simulink model "sl_ploop_test"  (R2022a)
settings: Solver=ode15s  StartTime=0.0  StopTime=1  RelTol=1e-3  EnableMultiTasking=on
PreLoadFcn:
  | G = 107.815;
InitFcn:
  | G = 107.815;
libraries: roblocks x1, robotcorelib x1
Description:
  | Test harness for position control loop with
  | trapezoidal trajectory.
  | 
  | Robotics, Vision and Control - 3rd Edition; Section 9.1.7
settings Model: Creator=pic  LastModifiedBy=rpill
settings SolverCC: AlgebraicLoopSolver=TrustRegion  MaxZcPerStep=1
settings DataIOCC: SaveFormat=Array  SignalLoggingSaveFormat=ModelDataLogs  TimeSaveName=t  OutputSaveName=y  OutputOption=SpecifiedOutputTimes  OutputTimes=[0:0.001:1]'
settings OptimizationCC: ExpressionDepthLimit=2147483647  LifeSpan=inf
settings DebuggingCC: UnderspecifiedInitializationDetection=Classic  MergeDetectMultiDrivingBlocksExec=none  SolverPrmCheckMsg=warning  UnconnectedInputMsg=warning  UnconnectedOutputMsg=warning  UnconnectedLineMsg=warning  AllowSymbolicDim=off  StateNameClashWarn=warning  SFUnexpectedBacktrackingDiag=warning  SFNoUnconditionalDefaultTransitionDiag=warning  SFExecutionAtInitializationDiag=none  SFMachineParentedDataDiag=warning  ArithmeticOperatorsInVariantConditions=warning
settings HardwareCC: ProdBitPerPointer=32  ProdBitPerSizeT=32  ProdBitPerPtrDiffT=32  ProdLargestAtomicFloat=None  ProdIntDivRoundTo=Undefined  ProdEndianess=Unspecified  ProdWordSize=32  ProdHWDeviceType=32-bit Generic
settings ModelReferenceCC: PropagateSignalLabelsOutOfModel=off
settings SFSimCC: SimUseLocalCustomCode=off  CustomCodeUndefinedFunction=UseInterfaceOnly
settings RTWCC: RTWUseLocalCustomCode=off
settings CodeAppCC: StateflowObjectComments=on
settings GRTTargetCC: TargetLangStandard=C89/C90 (ANSI)  CombineOutputUpdateFcns=off  GRTInterface=on
settings ConfigComp: CovMetricSettings=dw  CovSaveCumulativeToWorkspaceVar=on  CovSaveSingleToWorkspaceVar=on  CovExternalEMLEnable=off  CovSFcnEnable=off

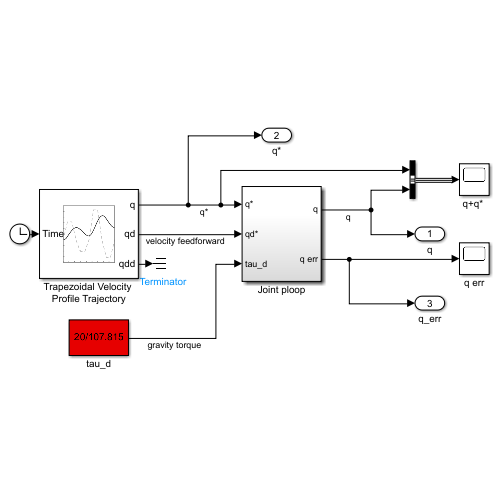
[thumbnail: Simulink's stored preview of the top-level diagram]
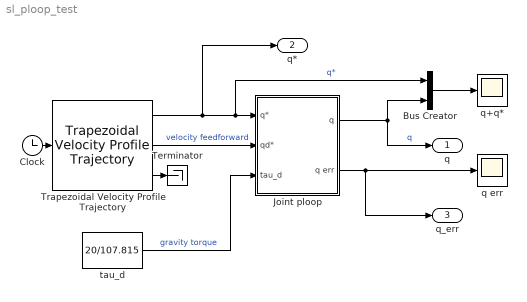
== system sl_ploop_test ==
  Bus Creator : BusCreator  Inputs=2
  Clock : Clock
  Joint ploop : Subsystem
  Terminator : Terminator
  Trapezoidal Velocity Profile Trajectory : robotcorelib/Trapezoidal Velocity Profile Trajectory  WaypointSource=Internal  Waypoints=[0 1]  NumParams=1  Parameter1=End Time  Parameter2=End Time  ParameterSource=Internal  PeakVelocity=[ 2; 2 ]  Acceleration=[ 1; 2 ]  EndTime=[1]  AccelTime=[ 1; 2 ]  SimulateUsing=Interpreted execution
      settings: SourceProductBaseCode=RO,NV,RR,UV
  q err : Scope
  "q+q* " : Scope
  tau_d : Constant  Value=20/107.815
  q : Outport  VectorParamsAs1DForOutWhenUnconnected=off
  q* : Outport  Port=2  VectorParamsAs1DForOutWhenUnconnected=off
  q_err : Outport  Port=3  VectorParamsAs1DForOutWhenUnconnected=off
  wires:
  Joint ploop/1(q) -> Bus Creator/2, q/1  "q"
  Joint ploop/2(q err) -> q_err/1, q err/1
  Trapezoidal Velocity Profile Trajectory/1 -> q*/1, Bus Creator/1, Joint ploop/1(q*)  "q*"
  tau_d/1 -> Joint ploop/3(tau_d)  "gravity torque"
  Trapezoidal Velocity Profile Trajectory/3 -> Terminator/1
  Trapezoidal Velocity Profile Trajectory/2 -> Joint ploop/2(qd*)  "velocity feedforward"
  Bus Creator/1 -> "q+q* "/1
  Clock/1 -> Trapezoidal Velocity Profile Trajectory/1

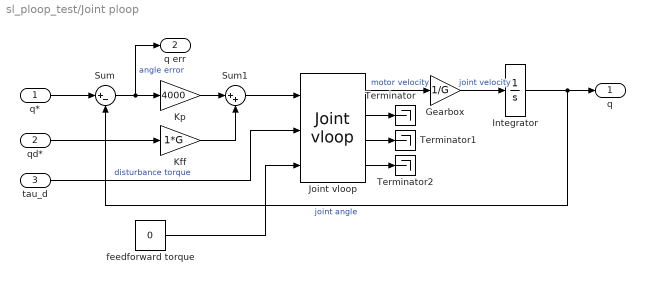
== system sl_ploop_test/Joint ploop ==
  q* : Inport
  qd* : Inport  Port=2
  tau_d : Inport  Port=3
  Gearbox : Gain  Gain=1/G
  Integrator : Integrator
  Joint vloop : roblocks/Joint vloop  J=580e-6  B=817e-6  Km=0.228  tau_max=0.9  Kv=0.6  Ki=0  T=0.001
  Kff : Gain  Gain=1*G
  Kp : Gain  Gain=4000
  Sum : Sum  Inputs=|+-
  Sum1 : Sum  Inputs=|++
  Terminator : Terminator
  Terminator1 : Terminator
  Terminator2 : Terminator
  feedforward torque : Constant  Value=0
  q : Outport  VectorParamsAs1DForOutWhenUnconnected=off
  q err : Outport  Port=2  VectorParamsAs1DForOutWhenUnconnected=off
  wires:
  Sum/1 -> Kp/1, q err/1  "angle error"
  Integrator/1 -> q/1, Sum/2  "joint angle"
  q*/1 -> Sum/1
  Kp/1 -> Sum1/1
  Sum1/1 -> Joint vloop/1
  qd*/1 -> Kff/1
  Kff/1 -> Sum1/2
  Joint vloop/2 -> Terminator/1
  Joint vloop/3 -> Terminator1/1
  Joint vloop/4 -> Terminator2/1
  Joint vloop/1 -> Gearbox/1  "motor velocity"
  tau_d/1 -> Joint vloop/2  "disturbance torque"
  feedforward torque/1 -> Joint vloop/3
  Gearbox/1 -> Integrator/1  "joint velocity"
